simulink model "IntegratedSteamNetworkSimulation"  (R2022b)
settings: Solver=ode4  StartTime=0  StopTime=1000  FixedStep=0.5  MaxStep=1  MinStep=1e-3  EnableMultiTasking=on
values from neighbouring files (symbols this model uses):
  Attemp1_PB = 334.14047    [BoilerParam.m]
  Attemp1_RB = 332.70172955    [BoilerParam.m]
  Attemp2_PB = 426.4464    [BoilerParam.m]
  Attemp2_RB = 423.6721137    [BoilerParam.m]
  Attempflow_init = 0    [BoilerParam.m]
  Attempflow_SS = 11355    [BoilerParam.m]
  Attempflow_SSRB = 2.3*11355    (= 26116.5)    [BoilerParam.m]
  FG_flow_RB = 2.3*FGFlow_SS    (= 420210)    [BoilerParam.m]
  FGFlow_SS = 182700    [BoilerParam.m]
  hf = u(3)    [Boiler3.m]    (also in Boiler4.m; BoilerParam.m = 900000)
  phin = 6.21000008802327    (= 6.21000008802)    [BoilerParam.m]
  qfsteadystate = 73.2301    [BoilerParam.m]
  qfsteadystate2 = 31.5677    [BoilerParam.m]
  Qsteadystate = 1.374070083420811e+008    (= 137407008.342)    [BoilerParam.m]
  Qsteadystate2 = 5.9194e+007    (= 59194000)    [BoilerParam.m]
  TFG_out1_initPB = 432.2968    [BoilerParam.m]
  TFG_out1_initRB = 434.8845734    [BoilerParam.m]
  TFG_out2_initPB = 483.8618    [BoilerParam.m]
  TFG_out2_initRB = 486.31627357    [BoilerParam.m]
  TFG_out3_initPB = 543.7293    [BoilerParam.m]
  TFG_out3_initRB = 545.8638828    [BoilerParam.m]
  TFG_out4_initPB = 611.0105    [BoilerParam.m]
  TFG_out4_initRB = 612.6928895    [BoilerParam.m]
  TFG_out5_initPB = 684.8106    [BoilerParam.m]
  TFG_out5_initRB = 685.9654778    [BoilerParam.m]
  TFG_out6_initPB = 764.5389    [BoilerParam.m]
  TFG_out6_initRB = 765.12376925    [BoilerParam.m]
  Ts_out1_init_PB = 303.33953    [BoilerParam.m]
  Ts_out1_init_RB = 302.2065815    [BoilerParam.m]
  Ts_out2_init_PB = 334.14047    [BoilerParam.m]
  Ts_out2_init_RB = 332.70172955    [BoilerParam.m]
  Ts_out3_init_PB = 375.4672    [BoilerParam.m]
  Ts_out3_init_RB = 373.4655693    [BoilerParam.m]
  Ts_out4_init_PB = 426.4464    [BoilerParam.m]
  Ts_out4_init_RB = 423.6721137    [BoilerParam.m]
  Ts_out5_init_PB = 485.4202    [BoilerParam.m]
  Ts_out5_init_RB = 481.745302    [BoilerParam.m]
  Ts_out6_init_PB = 550.8115    [BoilerParam.m]
  Ts_out6_init_RB = 546.1691598    [BoilerParam.m]
  X0 = [106.953303000225 ... (first row only)    [BoilerParam.m]
  X02 = [39.2837325596915 ... (first row only)    [BoilerParam.m]
undefined symbols (not defined in the file or in its folder): Param, Param2, Param3, Param4, Param5, Param6
libraries: slpidlib x1
(part 2 of 2)

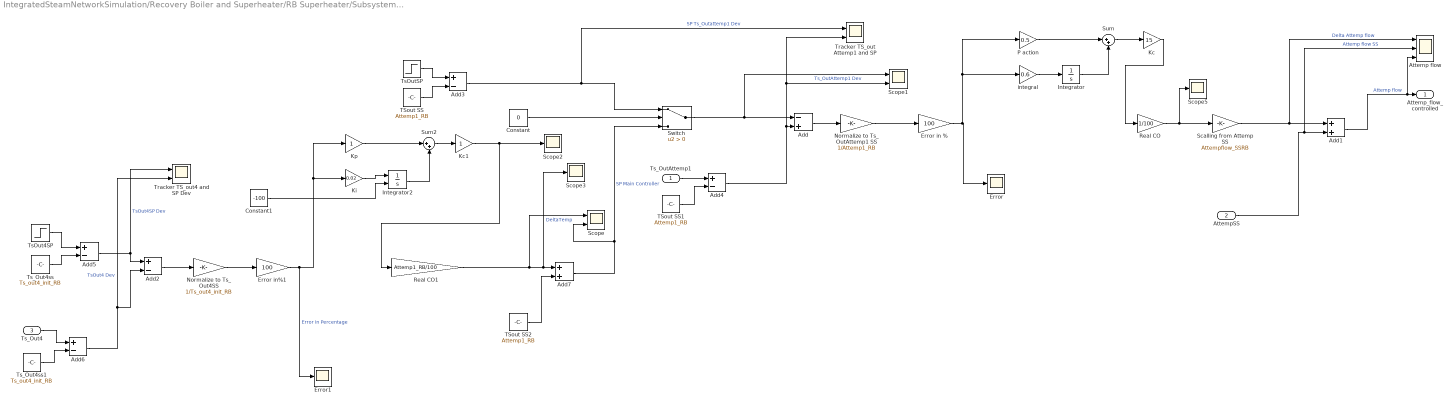
== system IntegratedSteamNetworkSimulation/Recovery Boiler and Superheater/RB Superheater/Subsystem1/Temperature Control2 ==
  Ts_OutAttemp1 : Inport
  AttempSS : Inport  Port=2
  Ts_Out4 : Inport  Port=3
  Add : Sum  Inputs=-+
  Add1 : Sum
  Add{2..6} (5 alike) : Sum  Inputs=+-
  Add7 : Sum
  Attemp flow : Scope  NumInputPorts=3
  Constant : Constant  Value=0
  Constant1 : Constant  Value=-100
  Error : Scope
  Error in % : Gain  Gain=100
  Error in%1 : Gain  Gain=100
  Error1 : Scope
  Integrator : Integrator
  Integrator2 : Integrator  InitialConditionSource=external  InitialCondition=-100.1
  Kc : Gain  Gain=15
  Kc1 : Gain
  Ki : Gain  Gain=0.02
  Kp : Gain
  Normalize to Ts_Out4SS : Gain  Gain=1/Ts_out4_init_RB
  Normalize to Ts_OutAttemp1 SS : Gain  Gain=1/Attemp1_RB
  P action : Gain  Gain=0.5
  Real CO : Gain  Gain=1/100
  Real CO1 : Gain  Gain=Attemp1_RB/100
  Scalling from Attemp SS : Gain  Gain=Attempflow_SSRB
  Scope : Scope  NumInputPorts=2
  Scope1 : Scope  NumInputPorts=2
  Scope2 : Scope
  Scope3 : Scope
  Scope5 : Scope
  Sum : Sum  Inputs=|++
  Sum2 : Sum  Inputs=|++
  Switch : Switch  Criteria=u2 > Threshold  SaturateOnIntegerOverflow=off  InputSameDT=off
  TSout SS : Constant  Value=Attemp1_RB
  TSout SS1 : Constant  Value=Attemp1_RB
  TSout SS2 : Constant  Value=Attemp1_RB
  Tracker TS_out Attemp1 and SP : Scope  NumInputPorts=2
  Tracker TS_out4 and SP Dev : Scope  NumInputPorts=2
  TsOut4SP : Step  Time=50000  Before=Ts_out4_init_RB  After=416  SampleTime=0
  TsOutSP : Step  Time=50  Before=Attemp1_RB  After=340  SampleTime=0
  Ts_Out4ss : Constant  Value=Ts_out4_init_RB
  Ts_Out4ss1 : Constant  Value=Ts_out4_init_RB
  integral : Gain  Gain=0.6
  Attemp_flow_controlled : Outport
  wires:
  Add1/1 -> Attemp flow/3, Attemp_flow_controlled/1  "Attemp flow"
  AttempSS/1 -> Attemp flow/2, Add1/2  "Attemp flow SS"
  TsOutSP/1 -> Add3/1
  TSout SS/1 -> Add3/2
  Ts_OutAttemp1/1 -> Add4/1
  TSout SS1/1 -> Add4/2
  Switch/1 -> Scope1/1, Add/1
  Add4/1 -> Tracker TS_out Attemp1 and SP/2, Scope1/2, Add/2  "Ts_OutAttemp1 Dev"
  Add3/1 -> Tracker TS_out Attemp1 and SP/1, Switch/1  "SP Ts_Outattemp1 Dev"
  Constant/1 -> Switch/2
  TsOut4SP/1 -> Add5/1
  Ts_Out4ss/1 -> Add5/2
  Add5/1 -> Tracker TS_out4 and SP Dev/1, Add2/1  "TsOut4SP Dev"
  Ts_Out4/1 -> Add6/1
  Ts_Out4ss1/1 -> Add6/2
  Add6/1 -> Add2/2, Tracker TS_out4 and SP Dev/2  "TsOut4 Dev"
  Real CO1/1 -> Scope/1, Add7/1, Scope3/1  "DeltaTemp"
  TSout SS2/1 -> Add7/2
  Add7/1 -> Scope/2, Switch/3  "SP Main Controller"
  Add/1 -> Normalize to Ts_OutAttemp1 SS/1
  Normalize to Ts_OutAttemp1 SS/1 -> Error in %/1
  Scalling from Attemp SS/1 -> Add1/1, Attemp flow/1  "Delta Attemp flow"
  Add2/1 -> Normalize to Ts_Out4SS/1
  Normalize to Ts_Out4SS/1 -> Error in%1/1
  Error in%1/1 -> Kp/1, Ki/1, Error1/1  "Error in Percentage"
  P action/1 -> Sum/1
  integral/1 -> Integrator/1
  Integrator/1 -> Sum/2
  Integrator2/1 -> Sum2/2
  Kp/1 -> Sum2/1
  Ki/1 -> Integrator2/1
  Constant1/1 -> Integrator2/2
  Error in %/1 -> P action/1, integral/1, Error/1
  Real CO/1 -> Scope5/1, Scalling from Attemp SS/1
  Sum/1 -> Kc/1
  Kc/1 -> Real CO/1
  Sum2/1 -> Kc1/1
  Kc1/1 -> Real CO1/1, Scope2/1

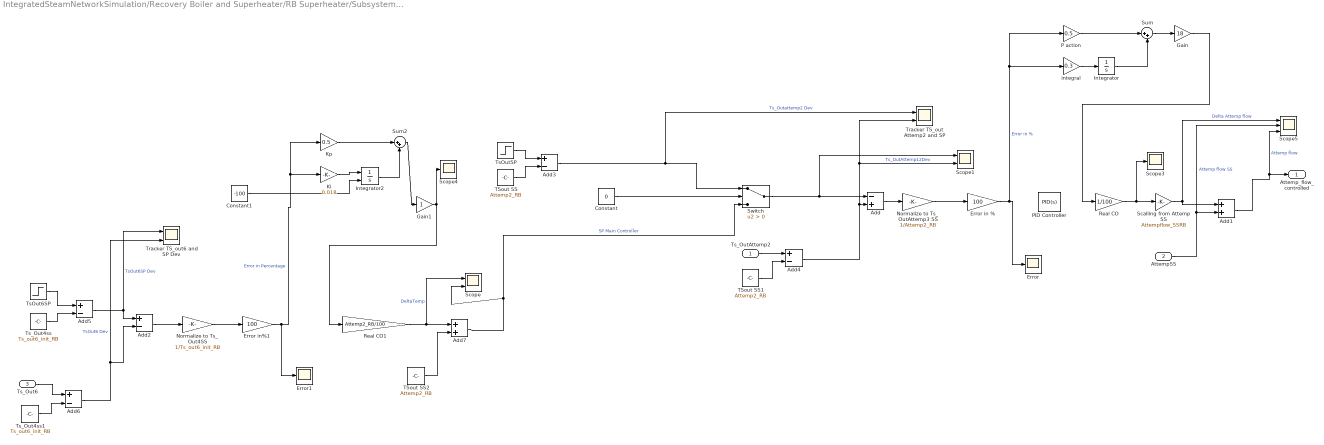
== system IntegratedSteamNetworkSimulation/Recovery Boiler and Superheater/RB Superheater/Subsystem2/Temperature Control ==
  Ts_OutAttemp2 : Inport
  AttempSS : Inport  Port=2
  Ts_Out6 : Inport  Port=3
  Add : Sum  Inputs=-+
  Add1 : Sum
  Add{2..6} (5 alike) : Sum  Inputs=+-
  Add7 : Sum
  Constant : Constant  Value=0
  Constant1 : Constant  Value=-100
  Error : Scope
  Error in % : Gain  Gain=100
  Error in%1 : Gain  Gain=100
  Error1 : Scope
  Gain : Gain  Gain=18
  Gain1 : Gain
  Integrator : Integrator
  Integrator2 : Integrator  InitialConditionSource=external  InitialCondition=-100.1
  Ki : Gain  Gain=0.018
  Kp : Gain  Gain=0.5
  Normalize to Ts_Out4SS : Gain  Gain=1/Ts_out6_init_RB
  Normalize to Ts_OutAttemp3 SS : Gain  Gain=1/Attemp2_RB
  P action : Gain  Gain=0.5
  PID Controller : slpidlib/PID Controller  Controller=PID  Form=Parallel  TimeDomain=Continuous-time  UseExternalTs=off  SampleTime=-1  IntegratorMethod=Forward Euler  FilterMethod=Forward Euler  ControllerParametersSource=internal  P=14.9271361165342  I=0.614463791653443  D=-137.003485064203  UseFilter=on  N=0.108954426301922  TunerSelectOption=Transfer Function Based (PID Tuner App)  InitialConditionSource=internal  InitialConditionForIntegrator=0  InitialConditionForFilter=0  DifferentiatorICPrevScaledInput=0  ExternalReset=none  TrackingMode=off  Kt=1  LimitOutput=off  SatLimitsSource=internal  UpperSaturationLimit=inf  LowerSaturationLimit=-inf  LinearizeAsGain=on  AntiWindupMode=none  Kb=1  POutMin=[]  POutMax=[]  IOutMin=[]  IOutMax=[]  DOutMin=[]  DOutMax=[]  NOutMin=[]  NOutMax=[]  SumOutMin=[]  SumOutMax=[]  SaturationOutMin=[]  SaturationOutMax=[]  PParamMin=[]  PParamMax=[]  IParamMin=[]  IParamMax=[]  DParamMin=[]  DParamMax=[]  NParamMin=[]  NParamMax=[]  KbParamMin=[]  KbParamMax=[]  KtParamMin=[]  KtParamMax=[]  KbOutMin=[]  KbOutMax=[]  KtOutMin=[]  KtOutMax=[]  IntegratorOutMin=[]  IntegratorOutMax=[]  FilterOutMin=[]  FilterOutMax=[]  SumI1OutMin=[]  SumI1OutMax=[]  SumI2OutMin=[]  SumI2OutMax=[]  SumI3OutMin=[]  SumI3OutMax=[]  SumI4OutMin=[]  SumI4OutMax=[]  SumDOutMin=[]  SumDOutMax=[]  DifferentiatorOutMin=[]  DifferentiatorOutMax=[]  FilterDiffOutCoefMin=[]  FilterDiffOutCoefMax=[]  ReciprocalOutMin=[]  ReciprocalOutMax=[]  SumDenOutMin=[]  SumDenOutMax=[]  SumNumOutMin=[]  SumNumOutMax=[]  DivideOutMin=[]  DivideOutMax=[]  UdiffTsProdOutMin=[]  UdiffTsProdOutMax=[]  NTsProdOutMin=[]  NTsProdOutMax=[]  UintegralTsProdOutMin=[]  UintegralTsProdOutMax=[]  UngainTsProdOutMin=[]  UngainTsProdOutMax=[]  IntegratorContinuousStateAttributes=''  IntegratorStateMustResolveToSignalObject=off  IntegratorRTWStateStorageClass=Auto  FilterContinuousStateAttributes=''  FilterStateMustResolveToSignalObject=off  FilterRTWStateStorageClass=Auto  ParallelPVariant=InternalParameters  IdealPVariant=Disabled  IVariant=InternalParameters  DVariant=InternalParameters  IntegratorVariant=Continuous  SatVariant=Disabled  AWVariant=Passthrough  PCopyVariant=Disabled  TRVariant=Disabled  FdbkBlocksVariant=Forward  IdealPFdbkVariant=Disabled  SatFdbkVariant=Disabled  DerivativeFilterVariant=ContFilter  NVariant=InternalParameters  NCopyVariant=Disabled  FilterICVariant=InternalICsFilter  IntegratorICVariant=InternalICs  ExternalResetVariant=Disabled  TRSumVariant=Passthrough  SumFdbkVariant=Disabled  SumVariant=Sum_PID  TsampFilterVariant=InternalTs  TsampNgainVariant=Passthrough  TsampIntegralVariant=Passthrough  ExternalSaturationOutDataTypeStr=Inherit: Same as second input
  Real CO : Gain  Gain=1/100
  Real CO1 : Gain  Gain=Attemp2_RB/100
  Scalling from Attemp SS : Gain  Gain=Attempflow_SSRB
  Scope : Scope  NumInputPorts=2
  Scope1 : Scope  NumInputPorts=2
  Scope3 : Scope
  Scope4 : Scope
  Scope5 : Scope  NumInputPorts=3
  Sum : Sum  Inputs=|++
  Sum2 : Sum  Inputs=|++
  Switch : Switch  Criteria=u2 > Threshold  SaturateOnIntegerOverflow=off  InputSameDT=off
  TSout SS : Constant  Value=Attemp2_RB
  TSout SS1 : Constant  Value=Attemp2_RB
  TSout SS2 : Constant  Value=Attemp2_RB
  Tracker TS_out Attemp2 and SP : Scope  NumInputPorts=2
  Tracker TS_out6 and SP Dev : Scope  NumInputPorts=2
  TsOut6SP : Step  Time=50000  Before=Ts_out6_init_RB  After=540  SampleTime=0
  TsOutSP : Step  Time=50  Before=Attemp2_RB  After=460  SampleTime=0
  Ts_Out4ss : Constant  Value=Ts_out6_init_RB
  Ts_Out4ss1 : Constant  Value=Ts_out6_init_RB
  integral : Gain  Gain=0.3
  Attemp_flow_controlled : Outport
  wires:
  Normalize to Ts_Out4SS/1 -> Error in%1/1
  TsOutSP/1 -> Add3/1
  AttempSS/1 -> Scope5/2, Add1/2  "Attemp flow SS"
  Scalling from Attemp SS/1 -> Scope5/1, Add1/1  "Delta Attemp flow"
  Normalize to Ts_OutAttemp3 SS/1 -> Error in %/1
  Add7/1 -> Scope/2, Switch/3  "SP Main Controller"
  Add4/1 -> Tracker TS_out Attemp2 and SP/2, Scope1/2, Add/2  "Ts_OutAttemp12Dev"
  Add/1 -> Normalize to Ts_OutAttemp3 SS/1
  Add2/1 -> Normalize to Ts_Out4SS/1
  Error in %/1 -> Error/1, P action/1, integral/1  "Error in %"
  Switch/1 -> Scope1/1, Add/1
  TSout SS1/1 -> Add4/2
  Real CO1/1 -> Scope/1, Add7/1  "DeltaTemp"
  Add5/1 -> Tracker TS_out6 and SP Dev/1, Add2/1  "TsOut6SP Dev"
  Ts_Out4ss/1 -> Add5/2
  Ts_OutAttemp2/1 -> Add4/1
  Ts_Out4ss1/1 -> Add6/2
  Add3/1 -> Tracker TS_out Attemp2 and SP/1, Switch/1  "Ts_Outattemp2 Dev"
  TsOut6SP/1 -> Add5/1
  Constant/1 -> Switch/2
  Add1/1 -> Scope5/3, Attemp_flow_controlled/1  "Attemp flow"
  Error in%1/1 -> Kp/1, Ki/1, Error1/1  "Error in Percentage"
  TSout SS2/1 -> Add7/2
  Add6/1 -> Add2/2, Tracker TS_out6 and SP Dev/2  "TsOut6 Dev"
  Ts_Out6/1 -> Add6/1
  TSout SS/1 -> Add3/2
  Real CO/1 -> Scope3/1, Scalling from Attemp SS/1
  Constant1/1 -> Integrator2/2
  Ki/1 -> Integrator2/1
  Kp/1 -> Sum2/1
  Integrator2/1 -> Sum2/2
  integral/1 -> Integrator/1
  Integrator/1 -> Sum/2
  P action/1 -> Sum/1
  Sum/1 -> Gain/1
  Gain/1 -> Real CO/1
  Sum2/1 -> Gain1/1
  Gain1/1 -> Scope4/1, Real CO1/1

== system IntegratedSteamNetworkSimulation/Recovery Boiler and Superheater/Recovery Boiler/3 Element Level Control System/FB Level Control ==
  In1 : Inport
  In2 : Inport  Port=2
  1/Ti1 : Gain  Gain=1/11.5/60  SaturateOnIntegerOverflow=on  OutDataTypeStr=Inherit: Same as input  ParamDataTypeStr=Inherit: Same as input
  Bias : Constant  Value=50
  Integrator1 : Integrator
  Kc1 : Gain  Gain=0.64  SaturateOnIntegerOverflow=on  OutDataTypeStr=Inherit: Same as input  ParamDataTypeStr=Inherit: Same as input
  P action1 : Gain  SaturateOnIntegerOverflow=on  OutDataTypeStr=Inherit: Same as input  ParamDataTypeStr=Inherit: Same as input
  Sum1 : Sum  Inputs=|++  InputSameDT=on  SaturateOnIntegerOverflow=on  OutDataTypeStr=Inherit: Same as first input
  Sum2 : Sum  Inputs=|++  InputSameDT=on  SaturateOnIntegerOverflow=on  OutDataTypeStr=Inherit: Same as first input
  Sum4 : Sum  Inputs=|+-  InputSameDT=on  SaturateOnIntegerOverflow=on  OutDataTypeStr=Inherit: Same as first input
  error as % of Range : Gain  Gain=100/25  SaturateOnIntegerOverflow=on  OutDataTypeStr=Inherit: Same as input  ParamDataTypeStr=Inherit: Same as input
  Out1 : Outport
  wires:
  1/Ti1/1 -> Integrator1/1
  Sum1/1 -> Kc1/1
  P action1/1 -> Sum1/1
  Integrator1/1 -> Sum1/2
  error as % of Range/1 -> 1/Ti1/1, P action1/1
  Sum4/1 -> error as % of Range/1
  In1/1 -> Sum4/1
  In2/1 -> Sum4/2
  Kc1/1 -> Sum2/1
  Sum2/1 -> Out1/1
  Bias/1 -> Sum2/2

== system IntegratedSteamNetworkSimulation/Recovery Boiler and Superheater/Recovery Boiler/Recovery Boiler/Recovery Boiler ==
  In2 : Inport
  In3 : Inport  Port=2
  Add : Sum
  Add1 : Sum
  Q (heat input in Watts) : Scope
  Q Nominal (in Watts) : Step  Time=50  Before=Qsteadystate  After=Qsteadystate  SampleTime=0
  Recovery Boiler : Subsystem
      mask Display: disp('')
  Vsd (steam in the drum in m3) : Scope
  Vst (total volume of steam in m3) : Scope
  Vwd (Volume of water in the drum in m3) : Scope
  Vwt (total water in m3) : Scope
  ar (steam quality) : Scope
  feedwater (kg/s) : Scope
  hf (feed H in J/kg)) : Step  Time=50  Before=hf  After=hf  SampleTime=0
  l (RB level in m from the bottom of drum) : Scope
  "p (pressure in Pa) " : Scope
  qct (condensation flow in kg/s) : Scope
  qdc (downcomer flow in kg/s) : Scope
  qf (feedwater in kg/s) : Step  Time=100  Before=qfsteadystate  After=qfsteadystate  SampleTime=0
  qr (riser flow in kg/s) : Scope
  qs (steam flow in kg/s) : Scope
  Out2 : Outport
  Out1 : Outport  Port=2
  Out3 : Outport  Port=3
  Out4 : Outport  Port=4
  wires:
  hf (feed H in J/kg))/1 -> Recovery Boiler/3(In4)
  qf (feedwater in kg/s)/1 -> Add/2
  Q Nominal (in Watts)/1 -> Add1/2
  Add1/1 -> Recovery Boiler/2(In3), Q (heat input in Watts)/1
  Add/1 -> Recovery Boiler/1(In1), Out4/1, feedwater (kg/s)/1
  In3/1 -> Add1/1
  In2/1 -> Add/1
  Recovery Boiler/6(Out6) -> Vst (total volume of steam in m3)/1
  Recovery Boiler/10(Out10) -> qr (riser flow in kg/s)/1
  Recovery Boiler/9(Out9) -> qct (condensation flow in kg/s)/1
  Recovery Boiler/8(Out8) -> qdc (downcomer flow in kg/s)/1
  Recovery Boiler/7(Out7) -> Vwd (Volume of water in the drum in m3)/1
  Recovery Boiler/5(Out5) -> Out2/1, l (RB level in m from the bottom of drum)/1
  Recovery Boiler/4(Out4) -> Vsd (steam in the drum in m3)/1
  Recovery Boiler/3(Out3) -> ar (steam quality)/1
  Recovery Boiler/2(Out2) -> "p (pressure in Pa) "/1, Out3/1
  Recovery Boiler/1(Out1) -> Vwt (total water in m3)/1
  Recovery Boiler/11(Out11) -> Out1/1, qs (steam flow in kg/s)/1

== system IntegratedSteamNetworkSimulation/Power Boiler and Superheater/Power Boiler/Power Boiler/Power Boiler/Power Boiler ==
  In1 : Inport
  In3 : Inport  Port=2
  In4 : Inport  Port=3
  Demux : Demux  Outputs=11
      settings: DisplayOption=none
  Mux : Mux  Inputs=3
  Power Boiler : S-Function  FunctionName=Boiler4  Parameters=Param2,X02  SFunctionDeploymentMode=off  EnableBusSupport=off
  Out1 : Outport
  Out2 : Outport  Port=2
  Out3 : Outport  Port=3
  Out4 : Outport  Port=4
  Out5 : Outport  Port=5
  Out6 : Outport  Port=6
  Out7 : Outport  Port=7
  Out8 : Outport  Port=8
  Out9 : Outport  Port=9
  Out10 : Outport  Port=10
  Out11 : Outport  Port=11
  wires:
  Mux/1 -> Power Boiler/1
  Power Boiler/1 -> Demux/1
  Demux/1 -> Out1/1
  Demux/2 -> Out2/1
  Demux/3 -> Out3/1
  In1/1 -> Mux/1
  Demux/4 -> Out4/1
  Demux/5 -> Out5/1
  Demux/6 -> Out6/1
  Demux/7 -> Out7/1
  Demux/8 -> Out8/1
  In4/1 -> Mux/3
  Demux/9 -> Out9/1
  Demux/10 -> Out10/1
  In3/1 -> Mux/2
  Demux/11 -> Out11/1

== system IntegratedSteamNetworkSimulation/Recovery Boiler and Superheater/Recovery Boiler/Recovery Boiler/Recovery Boiler/Recovery Boiler ==
  In1 : Inport
  In3 : Inport  Port=2
  In4 : Inport  Port=3
  Demux : Demux  Outputs=11
      settings: DisplayOption=none
  Mux : Mux  Inputs=3
  Recovery Boiler : S-Function  FunctionName=Boiler3  Parameters=Param,X0  SFunctionDeploymentMode=off  EnableBusSupport=off
  Out1 : Outport
  Out2 : Outport  Port=2
  Out3 : Outport  Port=3
  Out4 : Outport  Port=4
  Out5 : Outport  Port=5
  Out6 : Outport  Port=6
  Out7 : Outport  Port=7
  Out8 : Outport  Port=8
  Out9 : Outport  Port=9
  Out10 : Outport  Port=10
  Out11 : Outport  Port=11
  wires:
  Mux/1 -> Recovery Boiler/1
  Recovery Boiler/1 -> Demux/1
  Demux/1 -> Out1/1
  Demux/2 -> Out2/1
  Demux/3 -> Out3/1
  Demux/4 -> Out4/1
  In1/1 -> Mux/1
  Demux/5 -> Out5/1
  Demux/6 -> Out6/1
  In4/1 -> Mux/3
  Demux/7 -> Out7/1
  Demux/8 -> Out8/1
  Demux/9 -> Out9/1
  Demux/10 -> Out10/1
  In3/1 -> Mux/2
  Demux/11 -> Out11/1
